simulink model "mrefrobotarm_modified_previous_y_previous_u_previous_ref_pert_2"  (R2018b)
settings: Solver=FixedStepAuto  StartTime=0.0  StopTime=60  RelTol=1e-3  AbsTol=1e-6
undefined symbols (not defined in the file or in its folder): cc, options
libraries: neural x858, simulink x1
(part 28 of 32)

== system mrefrobotarm_modified_previous_y_previous_u_previous_ref_pert_2/m=0.01 sd =0.01/Layer 3/Delays 1 ==
  "p{3}" : Inport  PortDimensions=30
      mask Display: e = 0.06;c1 = [120 230 180]/255;c2 = ([120 230 180]+0)/(256+128);c3 = ([120 230 180]+128)/(256+128);patch([0 1 1 0],[0 0 1 1],c1);patch([0 1 1 1-e 1-e 0+e],[0 0 1 1-e 0+e 0+e],c2);patch([0 0 1 1-e 0+e 0+e],[0 1 1 1-e 1-e 0+e],c3);plot([0 1 1 0 0],[0 0 1 1 0]);
  mux : Mux  Inputs=1
      mask Display: e = 0.06;c1 = [120 150 230]/255;c2 = ([120 150 230]+0)/383;c3 = ([120 150 230]+128)/383;patch([0 1 1 0],[0 0 1 1],c1);patch([0 1 1 1-e 1-e 0+e],[0 0 1 1-e 0+e 0+e],c2);patch([0 0 1 1-e 0+e 0+e],[0 1 1 1-e 1-e 0+e],c3);plot([0 1 1 0 0],[0 0 1 1 0]);disp('Mux')
  "pd{3,2}" : Outport
      mask Display: e = 0.06;c1 = [120 230 180]/255;c2 = ([120 230 180]+0)/(256+128);c3 = ([120 230 180]+128)/(256+128);patch([0 1 1 0],[0 0 1 1],c1);patch([0 1 1 1-e 1-e 0+e],[0 0 1 1-e 0+e 0+e],c2);patch([0 0 1 1-e 0+e 0+e],[0 1 1 1-e 1-e 0+e],c3);plot([0 1 1 0 0],[0 0 1 1 0]);
  wires:
  "p{3}"/1 -> mux/1
  mux/1 -> "pd{3,2}"/1

== system mrefrobotarm_modified_previous_y_previous_u_previous_ref_pert_2/m=0.01 sd =0.01/Layer 3/LW{3,2} ==
  "ad{3,2}" : Inport  PortDimensions=30
      mask Display: e = 0.06;c1 = [120 230 180]/255;c2 = ([120 230 180]+0)/(256+128);c3 = ([120 230 180]+128)/(256+128);patch([0 1 1 0],[0 0 1 1],c1);patch([0 1 1 1-e 1-e 0+e],[0 0 1 1-e 0+e 0+e],c2);patch([0 0 1 1-e 0+e 0+e],[0 1 1 1-e 1-e 0+e],c3);plot([0 1 1 0 0],[0 0 1 1 0]);
  "IW{3,2}(1,:)'" : Constant  Value=[0.0028381381201219024745796559727750718593597412109375;-0.00708260609535531389380214051243456196971237659454345703125;-0.00583488335220346855669593111315407440997660160064697265625;0.01020530930108067869943599959015045897103846073150634765625;0.0035026247420214058798937362126935113337822258472442626953125;0.007372665491954556553355626391521582263521850109100341796875;0.0082512842468972780185509918737807311117649078369140625;-0.006754245741655124334046345069282324402593076229095458984375;0.001683452101721956591096063249324288335628807544708251953125;-0.00690829099421421365112561119303791201673448085784912109375;0.01314880348478297822367721892078407108783721923828125;-0.007470263091506845927469715462621024926193058490753173828125;-0.00542419932097103381363201179965471965260803699493408203125;-0.01146260049752216743368382623202705872245132923126220703125;-0.009116602607925426704493787610772415064275264739990234375;-0.0032803912590090062058323372440327148069627583026885986328125;-0.006661633151908582205213971150215002126060426235198974609375;-0.0289839272926558366716420778175233863294124603271484375;0.007080157965975715332607176577539576101116836071014404296875;1.106395796742202453089021219057030975818634033203125;0.0098157682894019597508172836342055234126746654510498046875;-0.00914110666628639191577665457089096889831125736236572265625;-0.00060787204210546621867272687467220748658291995525360107421875;-0.00883143986489790498717322719812727882526814937591552734375;0.0082676478536601351321255748416660935617983341217041015625;-0.00932936505581516591079083156046181102283298969268798828125;-0.00127195106162408637373584241458956967107951641082763671875;-0.00692592170297301294723535391995028476230800151824951171875;0.009542106880190574791367197349245543591678142547607421875;-0.00879287702148130560775296515885202097706496715545654296875]
      mask Display: e = 0.06;c1 = [120 150 230]/255;c2 = ([120 150 230]+0)/383;c3 = ([120 150 230]+128)/383;patch([0 1 1 0],[0 0 1 1],c1);patch([0 1 1 1-e 1-e 0+e],[0 0 1 1-e 0+e 0+e],c2);patch([0 0 1 1-e 0+e 0+e],[0 1 1 1-e 1-e 0+e],c3);plot([0 1 1 0 0],[0 0 1 1 0]);disp('weights');
  Mux : Mux  Inputs=1
      mask Display: e = 0.06;c1 = [120 150 230]/255;c2 = ([120 150 230]+0)/383;c3 = ([120 150 230]+128)/383;patch([0 1 1 0],[0 0 1 1],c1);patch([0 1 1 1-e 1-e 0+e],[0 0 1 1-e 0+e 0+e],c2);patch([0 0 1 1-e 0+e 0+e],[0 1 1 1-e 1-e 0+e],c3);plot([0 1 1 0 0],[0 0 1 1 0]);disp('Mux');
  dotprod1 : neural/Weight Functions/dotprod
  "lz{3,2}" : Outport
      mask Display: e = 0.06;c1 = [120 230 180]/255;c2 = ([120 230 180]+0)/(256+128);c3 = ([120 230 180]+128)/(256+128);patch([0 1 1 0],[0 0 1 1],c1);patch([0 1 1 1-e 1-e 0+e],[0 0 1 1-e 0+e 0+e],c2);patch([0 0 1 1-e 0+e 0+e],[0 1 1 1-e 1-e 0+e],c3);plot([0 1 1 0 0],[0 0 1 1 0]);
  wires:
  "IW{3,2}(1,:)'"/1 -> dotprod1/1
  "ad{3,2}"/1 -> dotprod1/2
  dotprod1/1 -> Mux/1
  Mux/1 -> "lz{3,2}"/1

== system mrefrobotarm_modified_previous_y_previous_u_previous_ref_pert_2/m=0.01 sd=0.001/Layer 1/Delays 1 ==
  "p{1}" : Inport  PortDimensions=10
      mask Display: e = 0.06;c1 = [120 230 180]/255;c2 = ([120 230 180]+0)/(256+128);c3 = ([120 230 180]+128)/(256+128);patch([0 1 1 0],[0 0 1 1],c1);patch([0 1 1 1-e 1-e 0+e],[0 0 1 1-e 0+e 0+e],c2);patch([0 0 1 1-e 0+e 0+e],[0 1 1 1-e 1-e 0+e],c3);plot([0 1 1 0 0],[0 0 1 1 0]);
  mux : Mux  Inputs=1
      mask Display: e = 0.06;c1 = [120 150 230]/255;c2 = ([120 150 230]+0)/383;c3 = ([120 150 230]+128)/383;patch([0 1 1 0],[0 0 1 1],c1);patch([0 1 1 1-e 1-e 0+e],[0 0 1 1-e 0+e 0+e],c2);patch([0 0 1 1-e 0+e 0+e],[0 1 1 1-e 1-e 0+e],c3);plot([0 1 1 0 0],[0 0 1 1 0]);disp('Mux')
  "pd{1,1}" : Outport
      mask Display: e = 0.06;c1 = [120 230 180]/255;c2 = ([120 230 180]+0)/(256+128);c3 = ([120 230 180]+128)/(256+128);patch([0 1 1 0],[0 0 1 1],c1);patch([0 1 1 1-e 1-e 0+e],[0 0 1 1-e 0+e 0+e],c2);patch([0 0 1 1-e 0+e 0+e],[0 1 1 1-e 1-e 0+e],c3);plot([0 1 1 0 0],[0 0 1 1 0]);
  wires:
  "p{1}"/1 -> mux/1
  mux/1 -> "pd{1,1}"/1

== system mrefrobotarm_modified_previous_y_previous_u_previous_ref_pert_2/m=0.01 sd=0.001/Layer 1/IW{1,1} ==
  "pd{1,1}" : Inport  PortDimensions=10
      mask Display: e = 0.06;c1 = [120 230 180]/255;c2 = ([120 230 180]+0)/(256+128);c3 = ([120 230 180]+128)/(256+128);patch([0 1 1 0],[0 0 1 1],c1);patch([0 1 1 1-e 1-e 0+e],[0 0 1 1-e 0+e 0+e],c2);patch([0 0 1 1-e 0+e 0+e],[0 1 1 1-e 1-e 0+e],c3);plot([0 1 1 0 0],[0 0 1 1 0]);
  "IW{1,1}(1,:)'" : Constant  Value=[-0.53323189650910762793500907719135284423828125;-0.35617407999863981427068893026444129645824432373046875;-0.843161425632632077764583300449885427951812744140625;0.187093228613186945974433683659299276769161224365234375;0.788926847723815161117499883403070271015167236328125;-0.388586419612412858892724898396409116685390472412109375;-0.242730084669846746248111912791500799357891082763671875;0.60821209125416064722458031610585749149322509765625;0.58996513988065457656517764917225576937198638916015625;-0.52937737680494567626965363160707056522369384765625]
      mask Display: e = 0.06;c1 = [120 150 230]/255;c2 = ([120 150 230]+0)/383;c3 = ([120 150 230]+128)/383;patch([0 1 1 0],[0 0 1 1],c1);patch([0 1 1 1-e 1-e 0+e],[0 0 1 1-e 0+e 0+e],c2);patch([0 0 1 1-e 0+e 0+e],[0 1 1 1-e 1-e 0+e],c3);plot([0 1 1 0 0],[0 0 1 1 0]);disp('Weights');
  "IW{1,1}(10,:)'" : Constant  Value=[1.0601630698805164509934684247127734124660491943359375;0.2151412306819258379864123753577587194740772247314453125;-0.56442326951252430600192155907279811799526214599609375;-0.6407765852799987005283810503897257149219512939453125;0.1813287044583277440867874474861309863626956939697265625;-1.142610587778535968794813015847466886043548583984375;1.026552167671368476220550292055122554302215576171875;-0.030083691716655723558115909099797136150300502777099609375;-0.65786528364150154146727800252847373485565185546875;-0.912102495887104236516051969374530017375946044921875]
      mask Display: e = 0.06;c1 = [120 150 230]/255;c2 = ([120 150 230]+0)/383;c3 = ([120 150 230]+128)/383;patch([0 1 1 0],[0 0 1 1],c1);patch([0 1 1 1-e 1-e 0+e],[0 0 1 1-e 0+e 0+e],c2);patch([0 0 1 1-e 0+e 0+e],[0 1 1 1-e 1-e 0+e],c3);plot([0 1 1 0 0],[0 0 1 1 0]);disp('Weights');
  "IW{1,1}(11,:)'" : Constant  Value=[0.06331086217247346159542331633929279632866382598876953125;-0.1907100691426644178960714270942844450473785400390625;0.71712643149386978702608530511497519910335540771484375;-0.572134877697007215857638584566302597522735595703125;0.98483505012747196705191754517727531492710113525390625;-1.227934973178955058159544933005236089229583740234375;0.303647608978811434088385112772812135517597198486328125;-0.15262908674143826903701892661047168076038360595703125;0.56165039275744010893731683609075844287872314453125;1.011042594486998513758635453996248543262481689453125]
      mask Display: e = 0.06;c1 = [120 150 230]/255;c2 = ([120 150 230]+0)/383;c3 = ([120 150 230]+128)/383;patch([0 1 1 0],[0 0 1 1],c1);patch([0 1 1 1-e 1-e 0+e],[0 0 1 1-e 0+e 0+e],c2);patch([0 0 1 1-e 0+e 0+e],[0 1 1 1-e 1-e 0+e],c3);plot([0 1 1 0 0],[0 0 1 1 0]);disp('Weights');
  "IW{1,1}(12,:)'" : Constant  Value=[0.3502232609861668510831123057869262993335723876953125;-0.9267993321065410849968202455784194171428680419921875;0.5108771945465988562062875644187442958354949951171875;0.0940273491361853785974744823761284351348876953125;0.2013117020597841866358379547818913124501705169677734375;-0.361790127989737142488735344159067608416080474853515625;1.0296392782657581843608340932405553758144378662109375;-0.50165161397467017412310497093130834400653839111328125;-0.83457176553406708929827573228976689279079437255859375;0.5640553552068487963566667531267739832401275634765625]
      mask Display: e = 0.06;c1 = [120 150 230]/255;c2 = ([120 150 230]+0)/383;c3 = ([120 150 230]+128)/383;patch([0 1 1 0],[0 0 1 1],c1);patch([0 1 1 1-e 1-e 0+e],[0 0 1 1-e 0+e 0+e],c2);patch([0 0 1 1-e 0+e 0+e],[0 1 1 1-e 1-e 0+e],c3);plot([0 1 1 0 0],[0 0 1 1 0]);disp('Weights');
  "IW{1,1}(13,:)'" : Constant  Value=[0.6146142254595357012902923088404349982738494873046875;0.253832160747340385142933882889337837696075439453125;-0.061773445638348752073643055382490274496376514434814453125;0.068905657699178612940471566616906784474849700927734375;-1.514976559026561364618146399152465164661407470703125;1.391177000052290058107473669224418699741363525390625;-0.1164684520114712407146129180546267889440059661865234375;0.39343633387243415189260531406034715473651885986328125;-0.503493266524980054299476250889711081981658935546875;-0.155393783188139622541967810320784337818622589111328125]
      mask Display: e = 0.06;c1 = [120 150 230]/255;c2 = ([120 150 230]+0)/383;c3 = ([120 150 230]+128)/383;patch([0 1 1 0],[0 0 1 1],c1);patch([0 1 1 1-e 1-e 0+e],[0 0 1 1-e 0+e 0+e],c2);patch([0 0 1 1-e 0+e 0+e],[0 1 1 1-e 1-e 0+e],c3);plot([0 1 1 0 0],[0 0 1 1 0]);disp('Weights');
  "IW{1,1}(14,:)'" : Constant  Value=[-0.81003261172384222188469493630691431462764739990234375;-0.57018386103918616836239152689813636243343353271484375;-0.7145443386722358791729448057594709098339080810546875;-0.55292804111540616585074303657165728509426116943359375;0.155532176305047065145714668688015080988407135009765625;0.07398011319300866472925548578132293187081813812255859375;-0.5534132996336769139134048600681126117706298828125;-0.1513948995394982233175795727220247499644756317138671875;-0.2298680343747128984599470413741073571145534515380859375;-0.82267172399519428171998924881336279213428497314453125]
      mask Display: e = 0.06;c1 = [120 150 230]/255;c2 = ([120 150 230]+0)/383;c3 = ([120 150 230]+128)/383;patch([0 1 1 0],[0 0 1 1],c1);patch([0 1 1 1-e 1-e 0+e],[0 0 1 1-e 0+e 0+e],c2);patch([0 0 1 1-e 0+e 0+e],[0 1 1 1-e 1-e 0+e],c3);plot([0 1 1 0 0],[0 0 1 1 0]);disp('Weights');
  "IW{1,1}(15,:)'" : Constant  Value=[-0.91312172818289327747010020175366662442684173583984375;0.71172938865590207324629545837524347007274627685546875;0.6841115721457071696676166538964025676250457763671875;0.10474775203729162764698656928885611705482006072998046875;0.531711221124022248574192417436279356479644775390625;-2.26091777142214755969007455860264599323272705078125;1.2225134534144503906105683199712075293064117431640625;0.4350518719322515881486879152362234890460968017578125;-0.62029415579110869227719149421318434178829193115234375;-0.78129171904518190938659927269327454268932342529296875]
      mask Display: e = 0.06;c1 = [120 150 230]/255;c2 = ([120 150 230]+0)/383;c3 = ([120 150 230]+128)/383;patch([0 1 1 0],[0 0 1 1],c1);patch([0 1 1 1-e 1-e 0+e],[0 0 1 1-e 0+e 0+e],c2);patch([0 0 1 1-e 0+e 0+e],[0 1 1 1-e 1-e 0+e],c3);plot([0 1 1 0 0],[0 0 1 1 0]);disp('Weights');
  "IW{1,1}(16,:)'" : Constant  Value=[0.61653355747392535324280515851569361984729766845703125;-0.441457906326986615486163145760656334459781646728515625;1.075231351596135365156214902526699006557464599609375;0.8676673217860038089810359451803378760814666748046875;-0.01341986154929593159923495448992980527691543102264404296875;-0.61137250169744294936435835552401840686798095703125;-0.267823285463873350664698591572232544422149658203125;-0.466301162734728380510063061592518351972103118896484375;-0.5981298281466449484611302978009916841983795166015625;-0.037640759103726585677041072131032706238329410552978515625]
      mask Display: e = 0.06;c1 = [120 150 230]/255;c2 = ([120 150 230]+0)/383;c3 = ([120 150 230]+128)/383;patch([0 1 1 0],[0 0 1 1],c1);patch([0 1 1 1-e 1-e 0+e],[0 0 1 1-e 0+e 0+e],c2);patch([0 0 1 1-e 0+e 0+e],[0 1 1 1-e 1-e 0+e],c3);plot([0 1 1 0 0],[0 0 1 1 0]);disp('Weights');
  "IW{1,1}(17,:)'" : Constant  Value=[0.0013734401717953904908942064366783597506582736968994140625;-0.380915216519360610991640214706421829760074615478515625;-0.443014106245981531539968045763089321553707122802734375;-1.27845546600293147321281139738857746124267578125;0.82660117801893451261463496848591603338718414306640625;-0.26555033417008389040603333342005498707294464111328125;-0.750392170823142468094602008932270109653472900390625;0.08405262535612183227851090805415879003703594207763671875;0.653646816804384744870048962184228003025054931640625;0.075928004384283986905046504034544341266155242919921875]
      mask Display: e = 0.06;c1 = [120 150 230]/255;c2 = ([120 150 230]+0)/383;c3 = ([120 150 230]+128)/383;patch([0 1 1 0],[0 0 1 1],c1);patch([0 1 1 1-e 1-e 0+e],[0 0 1 1-e 0+e 0+e],c2);patch([0 0 1 1-e 0+e 0+e],[0 1 1 1-e 1-e 0+e],c3);plot([0 1 1 0 0],[0 0 1 1 0]);disp('Weights');
  "IW{1,1}(18,:)'" : Constant  Value=[-0.677075743765576998356436888570897281169891357421875;-0.37600415657815988712542321081855334341526031494140625;0.42487296390769646592389108263887465000152587890625;0.08242252785399332981608466752732056193053722381591796875;0.373181453681661168264582784104277379810810089111328125;-0.792402669080374710830483309109695255756378173828125;-0.77912672861104270705112639916478656232357025146484375;-0.35973388770895997623711082269437611103057861328125;-0.5888207930955700053488044432015158236026763916015625;0.1475692592346480036535893987093004398047924041748046875]
      mask Display: e = 0.06;c1 = [120 150 230]/255;c2 = ([120 150 230]+0)/383;c3 = ([120 150 230]+128)/383;patch([0 1 1 0],[0 0 1 1],c1);patch([0 1 1 1-e 1-e 0+e],[0 0 1 1-e 0+e 0+e],c2);patch([0 0 1 1-e 0+e 0+e],[0 1 1 1-e 1-e 0+e],c3);plot([0 1 1 0 0],[0 0 1 1 0]);disp('Weights');
  "IW{1,1}(19,:)'" : Constant  Value=[-0.1853431622490974983730183112129452638328075408935546875;-0.321511842007140280497168305373634211719036102294921875;0.91804893211692728538508845304022543132305145263671875;-0.55889737459099764205205929101794026792049407958984375;-0.441455820754550865014920191242708824574947357177734375;-1.327522815303058933977808919735252857208251953125;-0.56457767366330113834038684217375703155994415283203125;-0.109495658575592624828232146683149039745330810546875;0.3873177885305703060936366455280221998691558837890625;0.2348357757993392025408496692762128077447414398193359375]
      mask Display: e = 0.06;c1 = [120 150 230]/255;c2 = ([120 150 230]+0)/383;c3 = ([120 150 230]+128)/383;patch([0 1 1 0],[0 0 1 1],c1);patch([0 1 1 1-e 1-e 0+e],[0 0 1 1-e 0+e 0+e],c2);patch([0 0 1 1-e 0+e 0+e],[0 1 1 1-e 1-e 0+e],c3);plot([0 1 1 0 0],[0 0 1 1 0]);disp('Weights');
  "IW{1,1}(2,:)'" : Constant  Value=[0.322172456378540472687888041036785580217838287353515625;-0.4037464179925602802967432580771856009960174560546875;-0.46997044680968247387653491387027315795421600341796875;-0.73514310496422419216600019353791140019893646240234375;-0.87235963990971843173838351503945887088775634765625;0.712402111524384817897725952207110822200775146484375;0.76644277630021007130523003070265986025333404541015625;0.334472599068433018576484982986585237085819244384765625;-0.590608860958847348143763156258501112461090087890625;0.1430488679526773221351021447844686917960643768310546875]
      mask Display: e = 0.06;c1 = [120 150 230]/255;c2 = ([120 150 230]+0)/383;c3 = ([120 150 230]+128)/383;patch([0 1 1 0],[0 0 1 1],c1);patch([0 1 1 1-e 1-e 0+e],[0 0 1 1-e 0+e 0+e],c2);patch([0 0 1 1-e 0+e 0+e],[0 1 1 1-e 1-e 0+e],c3);plot([0 1 1 0 0],[0 0 1 1 0]);disp('Weights');
  "IW{1,1}(20,:)'" : Constant  Value=[0.382878057274236016649382463583606295287609100341796875;0.1209441522349474495978682853092323057353496551513671875;0.26303035397876917134141194765106774866580963134765625;1.022465426664073806506394248572178184986114501953125;1.1803816799192190512002298419247381389141082763671875;-0.6580730927730906731909499285393394529819488525390625;-0.0307368407327227137482150709502093377523124217987060546875;0.09033247788889352258845377718898816965520381927490234375;-0.8265345891852484694339864290668629109859466552734375;0.312682358082809030985771414634655229747295379638671875]
      mask Display: e = 0.06;c1 = [120 150 230]/255;c2 = ([120 150 230]+0)/383;c3 = ([120 150 230]+128)/383;patch([0 1 1 0],[0 0 1 1],c1);patch([0 1 1 1-e 1-e 0+e],[0 0 1 1-e 0+e 0+e],c2);patch([0 0 1 1-e 0+e 0+e],[0 1 1 1-e 1-e 0+e],c3);plot([0 1 1 0 0],[0 0 1 1 0]);disp('Weights');
  "IW{1,1}(21,:)'" : Constant  Value=[0.55004877074209213017041975035681389272212982177734375;0.62093448684292074091217727982439100742340087890625;-0.50228481061416108133244051714427769184112548828125;-0.6509483882542930199832653670455329120159149169921875;-0.06498858615165183094664058671696693636476993560791015625;-0.9167508258910113116968432223075069487094879150390625;0.37717304427560438551125798767316155135631561279296875;0.86222753241918648203778730021440424025058746337890625;0.905248034716990890302668049116618931293487548828125;0.6323434974671371389121077299932949244976043701171875]
      mask Display: e = 0.06;c1 = [120 150 230]/255;c2 = ([120 150 230]+0)/383;c3 = ([120 150 230]+128)/383;patch([0 1 1 0],[0 0 1 1],c1);patch([0 1 1 1-e 1-e 0+e],[0 0 1 1-e 0+e 0+e],c2);patch([0 0 1 1-e 0+e 0+e],[0 1 1 1-e 1-e 0+e],c3);plot([0 1 1 0 0],[0 0 1 1 0]);disp('Weights');
  "IW{1,1}(22,:)'" : Constant  Value=[-0.80999709965564214986244451210950501263141632080078125;0.96966764106788350119359165546484291553497314453125;0.8598650775583751570962931509711779654026031494140625;0.87562395081228172610821047783247195184230804443359375;-0.375000966181332551219185234003816731274127960205078125;1.051710926923564048962589367874898016452789306640625;-0.003476135307298675210241345467920837108977138996124267578125;-0.237621726105286923402815091321826912462711334228515625;0.1726272806838935469642137832124717533588409423828125;0.986343050850502667259434019797481596469879150390625]
      mask Display: e = 0.06;c1 = [120 150 230]/255;c2 = ([120 150 230]+0)/383;c3 = ([120 150 230]+128)/383;patch([0 1 1 0],[0 0 1 1],c1);patch([0 1 1 1-e 1-e 0+e],[0 0 1 1-e 0+e 0+e],c2);patch([0 0 1 1-e 0+e 0+e],[0 1 1 1-e 1-e 0+e],c3);plot([0 1 1 0 0],[0 0 1 1 0]);disp('Weights');
  "IW{1,1}(23,:)'" : Constant  Value=[-0.2970732595173204426686197621165774762630462646484375;-0.61082310862881772361987486874568276107311248779296875;1.3106301134881730430237212203792296350002288818359375;-0.1607147235381714001078989895177073776721954345703125;0.03528125529591939757434460034346557222306728363037109375;-0.419080632668082930791797480196692049503326416015625;0.13312510091624207841931593065964989364147186279296875;0.7466199938454580742330790599226020276546478271484375;0.53482134143223236666386810611584223806858062744140625;0.423526960347863579148253165840287692844867706298828125]
      mask Display: e = 0.06;c1 = [120 150 230]/255;c2 = ([120 150 230]+0)/383;c3 = ([120 150 230]+128)/383;patch([0 1 1 0],[0 0 1 1],c1);patch([0 1 1 1-e 1-e 0+e],[0 0 1 1-e 0+e 0+e],c2);patch([0 0 1 1-e 0+e 0+e],[0 1 1 1-e 1-e 0+e],c3);plot([0 1 1 0 0],[0 0 1 1 0]);disp('Weights');
  "IW{1,1}(24,:)'" : Constant  Value=[0.055528307830612293194416650976563687436282634735107421875;-0.56122959575896957939988851649104617536067962646484375;-0.19666040250789418308841050020419061183929443359375;0.60847258887585653486240744314272888004779815673828125;0.10125068150863249238913255112493061460554599761962890625;1.30630890879859773434645831002853810787200927734375;-0.941916492259249782392771521699614822864532470703125;-0.390388154843826773454651402062154375016689300537109375;-0.87722034048789143678703794648754410445690155029296875;0.521260415805213650486393817118369042873382568359375]
      mask Display: e = 0.06;c1 = [120 150 230]/255;c2 = ([120 150 230]+0)/383;c3 = ([120 150 230]+128)/383;patch([0 1 1 0],[0 0 1 1],c1);patch([0 1 1 1-e 1-e 0+e],[0 0 1 1-e 0+e 0+e],c2);patch([0 0 1 1-e 0+e 0+e],[0 1 1 1-e 1-e 0+e],c3);plot([0 1 1 0 0],[0 0 1 1 0]);disp('Weights');
  "IW{1,1}(25,:)'" : Constant  Value=[0.5903833234238080596156805768259800970554351806640625;-0.9886263166129776180923727224580943584442138671875;0.40163491545071838828562249545939266681671142578125;-0.3615607974246983769006646980415098369121551513671875;-0.8528873074745895177528609565342776477336883544921875;-0.255531996012963447117982695999671705067157745361328125;0.71348837085301963778505296431831084191799163818359375;-0.43837639634493263951497965535963885486125946044921875;-0.29501055621108063231616824850789271295070648193359375;-0.267514144793130126398494894601753912866115570068359375]
      mask Display: e = 0.06;c1 = [120 150 230]/255;c2 = ([120 150 230]+0)/383;c3 = ([120 150 230]+128)/383;patch([0 1 1 0],[0 0 1 1],c1);patch([0 1 1 1-e 1-e 0+e],[0 0 1 1-e 0+e 0+e],c2);patch([0 0 1 1-e 0+e 0+e],[0 1 1 1-e 1-e 0+e],c3);plot([0 1 1 0 0],[0 0 1 1 0]);disp('Weights');
  "IW{1,1}(26,:)'" : Constant  Value=[-0.63045559129850048396548345408518798649311065673828125;0.64286947368534164137798825322533957660198211669921875;0.306128190430459745652314040853525511920452117919921875;0.993661675650066467113674661959521472454071044921875;0.1151639924783857960033373046826454810798168182373046875;-0.3686200036599587281926915238727815449237823486328125;0.8377239432107941308203180597047321498394012451171875;0.84212564871109563124917940513114444911479949951171875;-0.3472520885404948298713634358136914670467376708984375;-0.55606217961332171650923328343196772038936614990234375]
      mask Display: e = 0.06;c1 = [120 150 230]/255;c2 = ([120 150 230]+0)/383;c3 = ([120 150 230]+128)/383;patch([0 1 1 0],[0 0 1 1],c1);patch([0 1 1 1-e 1-e 0+e],[0 0 1 1-e 0+e 0+e],c2);patch([0 0 1 1-e 0+e 0+e],[0 1 1 1-e 1-e 0+e],c3);plot([0 1 1 0 0],[0 0 1 1 0]);disp('Weights');
  "IW{1,1}(27,:)'" : Constant  Value=[-0.315769963019390476066661221921094693243503570556640625;-0.1987339317726826148913232827908359467983245849609375;-0.8848914158889016334796906448900699615478515625;-0.07750773976416051869176015998164075426757335662841796875;-0.90008719773983558720686914966790936887264251708984375;0.11953991527106498649057897409875295124948024749755859375;-0.7426968653100762818297653211629949510097503662109375;0.38878141375412089697505280128098092973232269287109375;0.93513154608939463852124163167900405824184417724609375;0.371485452432128104849340388682321645319461822509765625]
      mask Display: e = 0.06;c1 = [120 150 230]/255;c2 = ([120 150 230]+0)/383;c3 = ([120 150 230]+128)/383;patch([0 1 1 0],[0 0 1 1],c1);patch([0 1 1 1-e 1-e 0+e],[0 0 1 1-e 0+e 0+e],c2);patch([0 0 1 1-e 0+e 0+e],[0 1 1 1-e 1-e 0+e],c3);plot([0 1 1 0 0],[0 0 1 1 0]);disp('Weights');
  "IW{1,1}(28,:)'" : Constant  Value=[-0.23941986683410731995280684714089147746562957763671875;-0.567759964867592170634225112735293805599212646484375;-0.97461242007175741264290991239249706268310546875;-0.899103773699696962040661674109287559986114501953125;0.07220990657503083276491651076867128722369670867919921875;-0.378577671925674319464150130443158559501171112060546875;-0.12004672674648642072270376957021653652191162109375;0.30262485255269677697498309498769231140613555908203125;0.1436518077379462521303565836205962114036083221435546875;0.79580996602296771857965040908311493694782257080078125]
      mask Display: e = 0.06;c1 = [120 150 230]/255;c2 = ([120 150 230]+0)/383;c3 = ([120 150 230]+128)/383;patch([0 1 1 0],[0 0 1 1],c1);patch([0 1 1 1-e 1-e 0+e],[0 0 1 1-e 0+e 0+e],c2);patch([0 0 1 1-e 0+e 0+e],[0 1 1 1-e 1-e 0+e],c3);plot([0 1 1 0 0],[0 0 1 1 0]);disp('Weights');
  "IW{1,1}(29,:)'" : Constant  Value=[-0.387497882076272837093000589447910897433757781982421875;-0.24191886890595915016177741563296876847743988037109375;0.52621577299517563464092972935759462416172027587890625;-0.72713769975839459558386579374200664460659027099609375;-1.2798959762292254627169540981412865221500396728515625;0.329788167313515290235415022834786213934421539306640625;-0.77953874742988105150942601540009491145610809326171875;0.5833996197827249208245348199852742254734039306640625;-0.51841043170843159604288530317717231810092926025390625;-0.04515182506228680725524071704057860188186168670654296875]
      mask Display: e = 0.06;c1 = [120 150 230]/255;c2 = ([120 150 230]+0)/383;c3 = ([120 150 230]+128)/383;patch([0 1 1 0],[0 0 1 1],c1);patch([0 1 1 1-e 1-e 0+e],[0 0 1 1-e 0+e 0+e],c2);patch([0 0 1 1-e 0+e 0+e],[0 1 1 1-e 1-e 0+e],c3);plot([0 1 1 0 0],[0 0 1 1 0]);disp('Weights');
  "IW{1,1}(3,:)'" : Constant  Value=[-0.050933882316000177181702923689954332076013088226318359375;1.059212889494542952917299771797843277454376220703125;0.330619844375596994012767027015797793865203857421875;-0.60538873769748280384561667233356274664402008056640625;-0.98914451230985600549416858484619297087192535400390625;-0.297510075495723336214126675258739851415157318115234375;-0.2179988189493673456098576934891752898693084716796875;0.8630126063675420677867577978759072721004486083984375;-0.2306593926767712410264010713945026509463787078857421875;0.40961553162285879725601489553810097277164459228515625]
      mask Display: e = 0.06;c1 = [120 150 230]/255;c2 = ([120 150 230]+0)/383;c3 = ([120 150 230]+128)/383;patch([0 1 1 0],[0 0 1 1],c1);patch([0 1 1 1-e 1-e 0+e],[0 0 1 1-e 0+e 0+e],c2);patch([0 0 1 1-e 0+e 0+e],[0 1 1 1-e 1-e 0+e],c3);plot([0 1 1 0 0],[0 0 1 1 0]);disp('Weights');
  "IW{1,1}(30,:)'" : Constant  Value=[-0.8938896815544692397992321275523863732814788818359375;0.81734066112043290974753517730277962982654571533203125;-0.573431398094300437406900528003461658954620361328125;-0.181619493399693521240578775177709758281707763671875;0.4727731878590037961629377605277113616466522216796875;-1.1028668818131153184225468066870234906673431396484375;0.5886007729362165985520505273598246276378631591796875;0.43974372337304423741244363554869778454303741455078125;0.361777734317867250002365153704886324703693389892578125;0.047652177057567558782213978929576114751398563385009765625]
      mask Display: e = 0.06;c1 = [120 150 230]/255;c2 = ([120 150 230]+0)/383;c3 = ([120 150 230]+128)/383;patch([0 1 1 0],[0 0 1 1],c1);patch([0 1 1 1-e 1-e 0+e],[0 0 1 1-e 0+e 0+e],c2);patch([0 0 1 1-e 0+e 0+e],[0 1 1 1-e 1-e 0+e],c3);plot([0 1 1 0 0],[0 0 1 1 0]);disp('Weights');
  "IW{1,1}(4,:)'" : Constant  Value=[0.93321351268110674936906434595584869384765625;-0.5866830952366886009485824615694582462310791015625;0.7208784745795735471318721465650014579296112060546875;-0.8812213608372474471508439819444902241230010986328125;-0.0485033992019721915678331924937083385884761810302734375;-0.206356878341764804485336526340688578784465789794921875;0.16298847950487982405576303790439851582050323486328125;0.79311533315789495279801712968037463724613189697265625;-0.5517791838376682189704069969593547284603118896484375;0.03477843216721854258111079616355709731578826904296875]
      mask Display: e = 0.06;c1 = [120 150 230]/255;c2 = ([120 150 230]+0)/383;c3 = ([120 150 230]+128)/383;patch([0 1 1 0],[0 0 1 1],c1);patch([0 1 1 1-e 1-e 0+e],[0 0 1 1-e 0+e 0+e],c2);patch([0 0 1 1-e 0+e 0+e],[0 1 1 1-e 1-e 0+e],c3);plot([0 1 1 0 0],[0 0 1 1 0]);disp('Weights');
  "IW{1,1}(5,:)'" : Constant  Value=[-0.7556663162900465469107302851625718176364898681640625;0.9383269822557893657943850485025905072689056396484375;-0.8169796658057706384425955548067577183246612548828125;0.3372024549351799738161616915022023022174835205078125;0.7981524735493377153972005544346757233142852783203125;-0.69153416133776335339433671833830885589122772216796875;-0.0312478012429383521231240905535742058418691158294677734375;0.3741566887969705046401713843806646764278411865234375;-0.40576771046058812686396777280606329441070556640625;-0.706660885018375761745801355573348701000213623046875]
      mask Display: e = 0.06;c1 = [120 150 230]/255;c2 = ([120 150 230]+0)/383;c3 = ([120 150 230]+128)/383;patch([0 1 1 0],[0 0 1 1],c1);patch([0 1 1 1-e 1-e 0+e],[0 0 1 1-e 0+e 0+e],c2);patch([0 0 1 1-e 0+e 0+e],[0 1 1 1-e 1-e 0+e],c3);plot([0 1 1 0 0],[0 0 1 1 0]);disp('Weights');
  "IW{1,1}(6,:)'" : Constant  Value=[0.00098716743246830417242432265112483946722932159900665283203125;-0.89224081420098244610272786303539760410785675048828125;0.69160899471343062483441599397337995469570159912109375;-0.63108445909708377197233630795381031930446624755859375;-0.71266462745583292193174429485225118696689605712890625;0.1363199946804304618641623392250039614737033843994140625;0.5575494281974824328784734461805783212184906005859375;-0.7790888084490836806850211360142566263675689697265625;0.28326903187438612352622158141457475721836090087890625;0.54722892363609876298369272262789309024810791015625]
      mask Display: e = 0.06;c1 = [120 150 230]/255;c2 = ([120 150 230]+0)/383;c3 = ([120 150 230]+128)/383;patch([0 1 1 0],[0 0 1 1],c1);patch([0 1 1 1-e 1-e 0+e],[0 0 1 1-e 0+e 0+e],c2);patch([0 0 1 1-e 0+e 0+e],[0 1 1 1-e 1-e 0+e],c3);plot([0 1 1 0 0],[0 0 1 1 0]);disp('Weights');
  "IW{1,1}(7,:)'" : Constant  Value=[0.5604103823569677178539905071374960243701934814453125;0.374375101165851764672964918645448051393032073974609375;-0.1603619244909675334298526649945415556430816650390625;0.78938401448135853133436512507614679634571075439453125;0.7622343143011243160600542978500016033649444580078125;0.50436852970987489097609568489133380353450775146484375;-0.90709434980579783935894511159858666360378265380859375;0.5446525527449230796861456838087178766727447509765625;-0.604086395069142856328880952787585556507110595703125;-0.63940461316580832207279172507696785032749176025390625]
      mask Display: e = 0.06;c1 = [120 150 230]/255;c2 = ([120 150 230]+0)/383;c3 = ([120 150 230]+128)/383;patch([0 1 1 0],[0 0 1 1],c1);patch([0 1 1 1-e 1-e 0+e],[0 0 1 1-e 0+e 0+e],c2);patch([0 0 1 1-e 0+e 0+e],[0 1 1 1-e 1-e 0+e],c3);plot([0 1 1 0 0],[0 0 1 1 0]);disp('Weights');
  "IW{1,1}(8,:)'" : Constant  Value=[-0.022267550715628588176020485889239353127777576446533203125;-0.8571311152178024972414505100459791719913482666015625;-0.09676405899293698265051233420308562926948070526123046875;0.92851931426095435373468944817432202398777008056640625;0.5412887594861846007887606901931576430797576904296875;-0.428982192941566753408011436476954258978366851806640625;0.356691010107674955076362266481737606227397918701171875;-1.0073464288006233058325733509263955056667327880859375;-0.334307248446535976160731706841033883392810821533203125;-0.49947290779607822486241275328211486339569091796875]
      mask Display: e = 0.06;c1 = [120 150 230]/255;c2 = ([120 150 230]+0)/383;c3 = ([120 150 230]+128)/383;patch([0 1 1 0],[0 0 1 1],c1);patch([0 1 1 1-e 1-e 0+e],[0 0 1 1-e 0+e 0+e],c2);patch([0 0 1 1-e 0+e 0+e],[0 1 1 1-e 1-e 0+e],c3);plot([0 1 1 0 0],[0 0 1 1 0]);disp('Weights');
  "IW{1,1}(9,:)'" : Constant  Value=[-0.7805965342272174201099232959677465260028839111328125;-0.06300073013028140156421841311384923756122589111328125;0.30724110899166046095842830254696309566497802734375;0.1599988273400072824603768140150350518524646759033203125;-0.73675350489855062630084603370050899684429168701171875;-0.06383814943585520984559167345651076175272464752197265625;0.357127556437940418820886634421185590326786041259765625;-0.8678814315711289584243104400229640305042266845703125;0.5649763584866211996171614373452030122280120849609375;-0.416783761417174158925291749255848117172718048095703125]
      mask Display: e = 0.06;c1 = [120 150 230]/255;c2 = ([120 150 230]+0)/383;c3 = ([120 150 230]+128)/383;patch([0 1 1 0],[0 0 1 1],c1);patch([0 1 1 1-e 1-e 0+e],[0 0 1 1-e 0+e 0+e],c2);patch([0 0 1 1-e 0+e 0+e],[0 1 1 1-e 1-e 0+e],c3);plot([0 1 1 0 0],[0 0 1 1 0]);disp('Weights');
  Mux : Mux  Inputs=30
      mask Display: e = 0.06;c1 = [120 150 230]/255;c2 = ([120 150 230]+0)/383;c3 = ([120 150 230]+128)/383;patch([0 1 1 0],[0 0 1 1],c1);patch([0 1 1 1-e 1-e 0+e],[0 0 1 1-e 0+e 0+e],c2);patch([0 0 1 1-e 0+e 0+e],[0 1 1 1-e 1-e 0+e],c3);plot([0 1 1 0 0],[0 0 1 1 0]);disp('Mux');
  dotprod{1..30} (30 alike) : neural/Weight Functions/dotprod
  "iz{1,1}" : Outport
      mask Display: e = 0.06;c1 = [120 230 180]/255;c2 = ([120 230 180]+0)/(256+128);c3 = ([120 230 180]+128)/(256+128);patch([0 1 1 0],[0 0 1 1],c1);patch([0 1 1 1-e 1-e 0+e],[0 0 1 1-e 0+e 0+e],c2);patch([0 0 1 1-e 0+e 0+e],[0 1 1 1-e 1-e 0+e],c3);plot([0 1 1 0 0],[0 0 1 1 0]);
  wires:
  "IW{1,1}(1,:)'"/1 -> dotprod1/1
  "pd{1,1}"/1 -> dotprod1/2, dotprod2/2, dotprod3/2, dotprod4/2, dotprod5/2, dotprod6/2, dotprod7/2, dotprod8/2, dotprod9/2, dotprod10/2, dotprod11/2, dotprod12/2, dotprod13/2, dotprod14/2, dotprod15/2, dotprod16/2, dotprod17/2, dotprod18/2, dotprod19/2, dotprod20/2, dotprod21/2, dotprod22/2, dotprod23/2, dotprod24/2, dotprod25/2, dotprod26/2, dotprod27/2, dotprod28/2, dotprod29/2, dotprod30/2
  dotprod1/1 -> Mux/1
  "IW{1,1}(2,:)'"/1 -> dotprod2/1
  dotprod2/1 -> Mux/2
  "IW{1,1}(3,:)'"/1 -> dotprod3/1
  dotprod3/1 -> Mux/3
  "IW{1,1}(4,:)'"/1 -> dotprod4/1
  dotprod4/1 -> Mux/4
  "IW{1,1}(5,:)'"/1 -> dotprod5/1
  dotprod5/1 -> Mux/5
  "IW{1,1}(6,:)'"/1 -> dotprod6/1
  dotprod6/1 -> Mux/6
  "IW{1,1}(7,:)'"/1 -> dotprod7/1
  dotprod7/1 -> Mux/7
  "IW{1,1}(8,:)'"/1 -> dotprod8/1
  dotprod8/1 -> Mux/8
  "IW{1,1}(9,:)'"/1 -> dotprod9/1
  dotprod9/1 -> Mux/9
  "IW{1,1}(10,:)'"/1 -> dotprod10/1
  dotprod10/1 -> Mux/10
  "IW{1,1}(11,:)'"/1 -> dotprod11/1
  dotprod11/1 -> Mux/11
  "IW{1,1}(12,:)'"/1 -> dotprod12/1
  dotprod12/1 -> Mux/12
  "IW{1,1}(13,:)'"/1 -> dotprod13/1
  dotprod13/1 -> Mux/13
  "IW{1,1}(14,:)'"/1 -> dotprod14/1
  dotprod14/1 -> Mux/14
  "IW{1,1}(15,:)'"/1 -> dotprod15/1
  dotprod15/1 -> Mux/15
  "IW{1,1}(16,:)'"/1 -> dotprod16/1
  dotprod16/1 -> Mux/16
  "IW{1,1}(17,:)'"/1 -> dotprod17/1
  dotprod17/1 -> Mux/17
  "IW{1,1}(18,:)'"/1 -> dotprod18/1
  dotprod18/1 -> Mux/18
  "IW{1,1}(19,:)'"/1 -> dotprod19/1
  dotprod19/1 -> Mux/19
  "IW{1,1}(20,:)'"/1 -> dotprod20/1
  dotprod20/1 -> Mux/20
  "IW{1,1}(21,:)'"/1 -> dotprod21/1
  dotprod21/1 -> Mux/21
  "IW{1,1}(22,:)'"/1 -> dotprod22/1
  dotprod22/1 -> Mux/22
  "IW{1,1}(23,:)'"/1 -> dotprod23/1
  dotprod23/1 -> Mux/23
  "IW{1,1}(24,:)'"/1 -> dotprod24/1
  dotprod24/1 -> Mux/24
  "IW{1,1}(25,:)'"/1 -> dotprod25/1
  dotprod25/1 -> Mux/25
  "IW{1,1}(26,:)'"/1 -> dotprod26/1
  dotprod26/1 -> Mux/26
  "IW{1,1}(27,:)'"/1 -> dotprod27/1
  dotprod27/1 -> Mux/27
  "IW{1,1}(28,:)'"/1 -> dotprod28/1
  dotprod28/1 -> Mux/28
  "IW{1,1}(29,:)'"/1 -> dotprod29/1
  dotprod29/1 -> Mux/29
  "IW{1,1}(30,:)'"/1 -> dotprod30/1
  dotprod30/1 -> Mux/30
  Mux/1 -> "iz{1,1}"/1

== system mrefrobotarm_modified_previous_y_previous_u_previous_ref_pert_2/m=0.01 sd=0.001/Layer 2/Delays 1 ==
  "p{2}" : Inport  PortDimensions=30
      mask Display: e = 0.06;c1 = [120 230 180]/255;c2 = ([120 230 180]+0)/(256+128);c3 = ([120 230 180]+128)/(256+128);patch([0 1 1 0],[0 0 1 1],c1);patch([0 1 1 1-e 1-e 0+e],[0 0 1 1-e 0+e 0+e],c2);patch([0 0 1 1-e 0+e 0+e],[0 1 1 1-e 1-e 0+e],c3);plot([0 1 1 0 0],[0 0 1 1 0]);
  mux : Mux  Inputs=1
      mask Display: e = 0.06;c1 = [120 150 230]/255;c2 = ([120 150 230]+0)/383;c3 = ([120 150 230]+128)/383;patch([0 1 1 0],[0 0 1 1],c1);patch([0 1 1 1-e 1-e 0+e],[0 0 1 1-e 0+e 0+e],c2);patch([0 0 1 1-e 0+e 0+e],[0 1 1 1-e 1-e 0+e],c3);plot([0 1 1 0 0],[0 0 1 1 0]);disp('Mux')
  "pd{2,1}" : Outport
      mask Display: e = 0.06;c1 = [120 230 180]/255;c2 = ([120 230 180]+0)/(256+128);c3 = ([120 230 180]+128)/(256+128);patch([0 1 1 0],[0 0 1 1],c1);patch([0 1 1 1-e 1-e 0+e],[0 0 1 1-e 0+e 0+e],c2);patch([0 0 1 1-e 0+e 0+e],[0 1 1 1-e 1-e 0+e],c3);plot([0 1 1 0 0],[0 0 1 1 0]);
  wires:
  "p{2}"/1 -> mux/1
  mux/1 -> "pd{2,1}"/1
